simulink model "solar_tracker_SIL_plant"  (R2025b)
settings: Solver=ode4  StartTime=0  StopTime=60  FixedStep=0.01  RelTol=1e-3
settings Model: Creator=Kerem Bayer  LastModifiedBy=Kerem Bayer

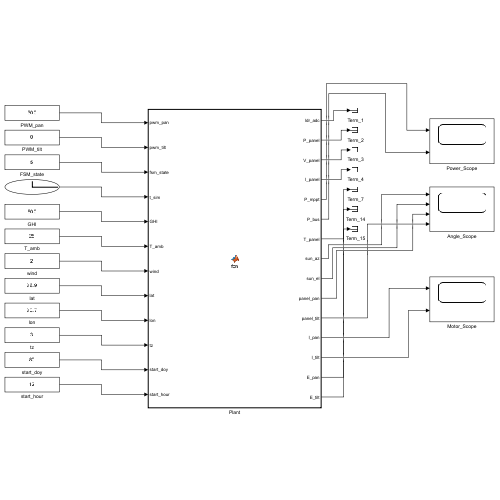
[thumbnail: Simulink's stored preview of the top-level diagram]
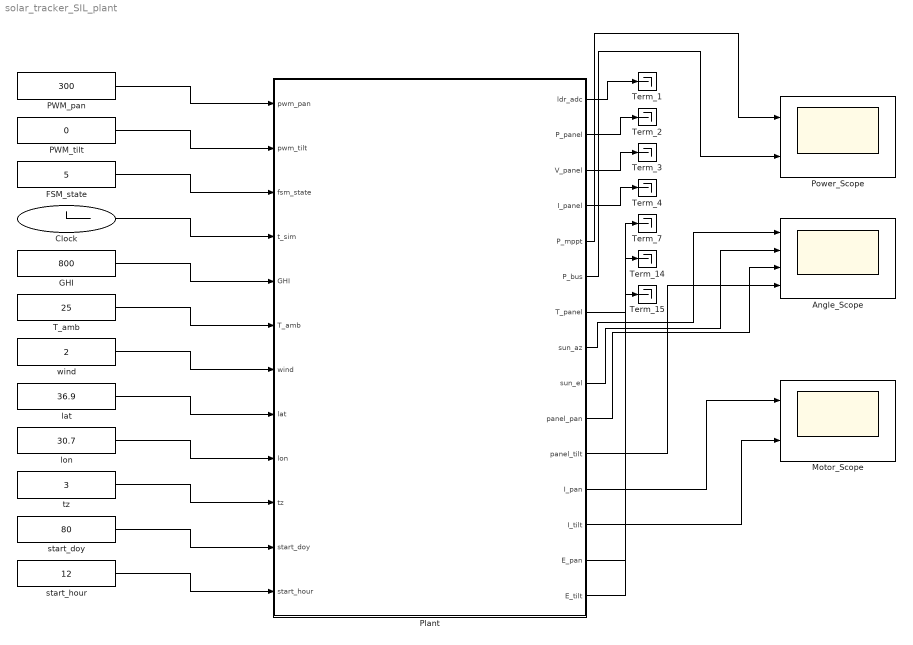
== system solar_tracker_SIL_plant ==
  Angle_Scope : Scope  NumInputPorts=4
      settings: ActiveDisplayYMinimum=-44.15703918318053  ActiveDisplayYMaximum=190.56668957130361
  Clock : Clock
  FSM_state : Constant  Value=5  OutDataTypeStr=uint8
  GHI : Constant  Value=800  OutDataTypeStr=double
  Motor_Scope : Scope  NumInputPorts=2
      settings: ActiveDisplayYMinimum=-0.60092183800125609  ActiveDisplayYMaximum=1.4590296251224235
  PWM_pan : Constant  Value=300  OutDataTypeStr=int16
  PWM_tilt : Constant  Value=0  OutDataTypeStr=int16
  Plant : MATLAB Function  TreatAsAtomicUnit=on
  Power_Scope : Scope  NumInputPorts=2
      settings: ActiveDisplayYMinimum=-4.2836309081746213  ActiveDisplayYMaximum=7.83290759655419
  T_amb : Constant  Value=25  OutDataTypeStr=double
  Term_{1..4,7,14..15} (7 alike) : Terminator
  lat : Constant  Value=36.9  OutDataTypeStr=double
  lon : Constant  Value=30.7  OutDataTypeStr=double
  start_doy : Constant  Value=80  OutDataTypeStr=double
  start_hour : Constant  Value=12  OutDataTypeStr=double
  tz : Constant  Value=3  OutDataTypeStr=double
  wind : Constant  Value=2  OutDataTypeStr=double
  wires:
  PWM_pan/1 -> Plant/1(pwm_pan)
  PWM_tilt/1 -> Plant/2(pwm_tilt)
  FSM_state/1 -> Plant/3(fsm_state)
  Clock/1 -> Plant/4(t_sim)
  GHI/1 -> Plant/5(GHI)
  T_amb/1 -> Plant/6(T_amb)
  wind/1 -> Plant/7(wind)
  lat/1 -> Plant/8(lat)
  lon/1 -> Plant/9(lon)
  tz/1 -> Plant/10(tz)
  start_doy/1 -> Plant/11(start_doy)
  start_hour/1 -> Plant/12(start_hour)
  Plant/5(P_mppt) -> Power_Scope/1
  Plant/6(P_bus) -> Power_Scope/2
  Plant/8(sun_az) -> Angle_Scope/1
  Plant/9(sun_el) -> Angle_Scope/2
  Plant/10(panel_pan) -> Angle_Scope/3
  Plant/11(panel_tilt) -> Angle_Scope/4
  Plant/12(I_pan) -> Motor_Scope/1
  Plant/13(I_tilt) -> Motor_Scope/2
  Plant/1(ldr_adc) -> Term_1/1
  Plant/2(P_panel) -> Term_2/1
  Plant/3(V_panel) -> Term_3/1
  Plant/4(I_panel) -> Term_4/1
  Plant/7(T_panel) -> Term_7/1
  Plant/14(E_pan) -> Term_14/1
  Plant/15(E_tilt) -> Term_15/1

== matlab function solar_tracker_SIL_plant/Plant ==
  data: pwm_pan input; ldr_adc output; pwm_tilt input; fsm_state input; t_sim input; GHI input; T_amb input; wind input; lat input; lon input; tz input; start_doy input; start_hour input; P_panel output; V_panel output; I_panel output; P_mppt output; P_bus output; T_panel output; sun_az output; sun_el output; panel_pan output; panel_tilt output; I_pan output; I_tilt output; E_pan output; E_tilt output
function [ldr_adc, P_panel, V_panel, I_panel, P_mppt, P_bus, ...
          T_panel, sun_az, sun_el, panel_pan, panel_tilt, ...
          I_pan, I_tilt, E_pan, E_tilt] = fcn( ...
          pwm_pan, pwm_tilt, fsm_state, t_sim, GHI, T_amb, wind, ...
          lat, lon, tz, start_doy, start_hour)
    coder.extrinsic('plant_step');

    %% Pre-declare outputs so Simulink can infer types
    ldr_adc    = uint16(zeros(1,4));
    P_panel    = zeros(4,1);
    V_panel    = zeros(4,1);
    I_panel    = zeros(4,1);
    T_panel    = zeros(4,1);
    P_mppt     = 0;   P_bus = 0;
    sun_az     = 0;   sun_el = 0;
    panel_pan  = 0;   panel_tilt = 0;
    I_pan      = 0;   I_tilt = 0;
    E_pan      = 0;   E_tilt = 0;

    [ldr_adc, P_panel, V_panel, I_panel, P_mppt, P_bus, ...
     T_panel, sun_az, sun_el, panel_pan, panel_tilt, ...
     I_pan, I_tilt, E_pan, E_tilt] = ...
         plant_step(pwm_pan, pwm_tilt, fsm_state, t_sim, ...
                    GHI, T_amb, wind, ...
                    lat, lon, tz, start_doy, start_hour);
end
